simulink model "untitled"  (Simulink 7.9)
settings: Solver=ode45  StartTime=0.0  StopTime=10.0  MaxStep=0.02  MinStep=0.01  RelTol=1e-3
libraries: simulink x1
settings Model: Creator=aziemba  LastModifiedBy=aziemba

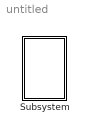
== system untitled ==
  Subsystem : Subsystem  mask{n=3, g=9.81, k=1, m=2, l=4, xi=[ -1 1 1], yi=[ 1  1 -1 ], di=[ 0.1 0.1 0.1 ], ai=[ 1 -1 1.5 ]}
      mask TabNameString: n,g,k,m,l,xi,yi,di,ai

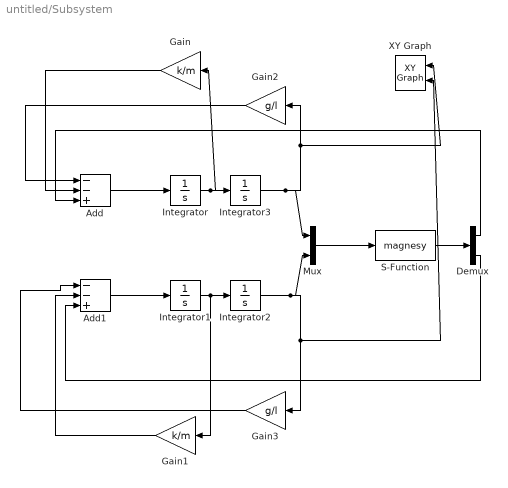
== system untitled/Subsystem ==
  Add : Sum  Inputs=--+
  Add1 : Sum  Inputs=--+
  Demux : Demux  Outputs=2
  Gain : Gain  Gain=k/m
  Gain1 : Gain  Gain=k/m
  Gain2 : Gain  Gain=g/l
  Gain3 : Gain  Gain=g/l
  Integrator : Integrator
  Integrator1 : Integrator
  Integrator2 : Integrator  InitialCondition=-1
  Integrator3 : Integrator  InitialCondition=-1
  Mux : Mux  Inputs=2
  S-Function : S-Function  FunctionName=magnesy  Parameters=ai,di,xi,yi  EnableBusSupport=off
  XY Graph : simulink/Sinks/XY Graph  xmin=-1  xmax=1  ymin=-1  ymax=1  st=-1
  wires:
  Integrator/1 -> Integrator3/1, Gain/1
  Integrator1/1 -> Integrator2/1, Gain1/1
  Add1/1 -> Integrator1/1
  Add/1 -> Integrator/1
  Integrator3/1 -> Mux/1, Gain2/1, XY Graph/1
  Integrator2/1 -> Mux/2, Gain3/1, XY Graph/2
  Mux/1 -> S-Function/1
  Demux/1 -> Add/3
  Demux/2 -> Add1/3
  S-Function/1 -> Demux/1
  Gain1/1 -> Add1/2
  Gain/1 -> Add/2
  Gain3/1 -> Add1/1
  Gain2/1 -> Add/1
